simulink model "SPNCS_example_wx_timer"  (R2022b)
settings: Solver=VariableStepAuto  StartTime=0.0  StopTime=T  MaxStep=MaxStep  RelTol=RelTol
values from neighbouring files (symbols this model uses):
  epsilon = 0.0014    [initialization.m]
  J = 100000000    [initialization.m]
  rule = 2    [initialization.m]
  T = 20    [initialization.m]
  tau_mati = epsilon*T_star    (= 0.00123088)    [initialization.m]
  tau_miati = tau_mati    (= 0.00123088)    [initialization.m]
  tau_s_mati = 0.1072    [initialization.m]
  tau_s_miati = 0.0029    [initialization.m]
  x0 = [10;-2;5;0;0;0;0;0]    [initialization.m]
undefined symbols (not defined in the file or in its folder): tau_f_mati, tau_f_miati
libraries: simulink x6
settings Model: Creator=weixuanw  LastModifiedBy=weixuanw
settings ModelReferenceCC: EnableRefExpFcnMdlSchedulingChecks=on

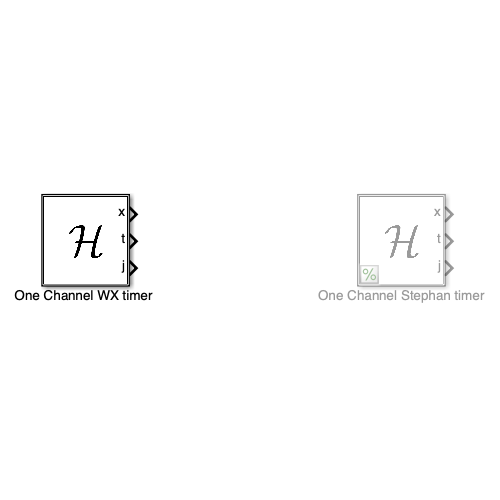
[thumbnail: Simulink's stored preview of the top-level diagram]
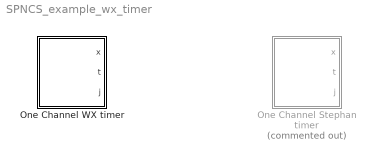
== system SPNCS_example_wx_timer ==
  One Channel Stephan timer : Subsystem  Commented=on  LoadFcn=set_param(gcb,'LinkStatus','none')
      settings: CopyFcn=|
      | set_param(gcb,'LinkStatus','none'),
      | set_param(gcs, 'MaxStep', 'MaxStep', 'RelTol', 'RelTol','Stop time', 'T')
      mask Display:
      | image(imread('Hcal.jpg'))
      | %plot([5 20 20 5 5],[5 5 20 20 5])
      | %text(8,13,'HyEq_mdl')
      | port_label('output', 1, 'x')
      | port_label('output', 2, 't')
      | port_label('output', 3, 'j')
  "One Channel WX timer " : Subsystem  LoadFcn=set_param(gcb,'LinkStatus','none')
      settings: CopyFcn=|
      | set_param(gcb,'LinkStatus','none'),
      | set_param(gcs, 'MaxStep', 'MaxStep', 'RelTol', 'RelTol','Stop time', 'T')
      mask Display:
      | image(imread('Hcal.jpg'))
      | %plot([5 20 20 5 5],[5 5 20 20 5])
      | %text(8,13,'HyEq_mdl')
      | port_label('output', 1, 'x')
      | port_label('output', 2, 't')
      | port_label('output', 3, 'j')

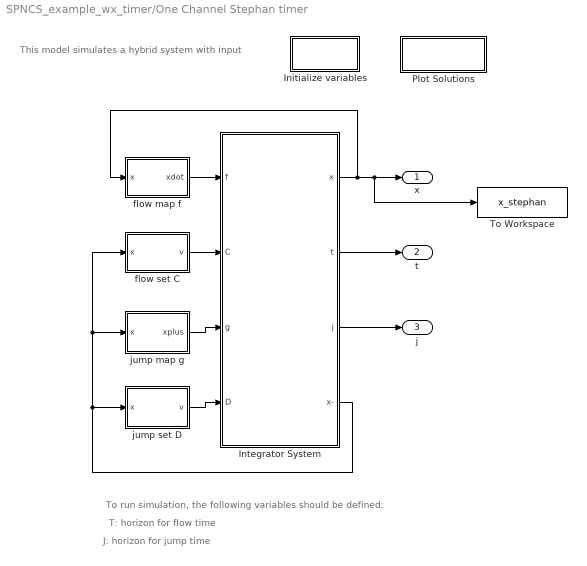
== system SPNCS_example_wx_timer/One Channel Stephan timer ==
  note: J: horizon for jump time
  note: T: horizon for flow time
  note: To run simulation, the following variables should be defined:
  note: This model simulates a hybrid system with input
  Initialize variables : Subsystem  Priority=-10
      settings: OpenFcn=|
      | try
      |      clearvars -except inifile pathfile_in pathfile_pos posfile
      |      cd(pathfile_in);
      |      eval(inifile);
      | catch
      |      [inifile,pathfile_in] = getInitializationfile;
      |      cd(pathfile_in);
      |      inifile = strrep(inifile,'.m','');
      |      eval(inifile);
      | end
      mask Display: disp('Double Click\n to Initialize')
  Integrator System : Subsystem  Priority=2  mask(Hybrid Integrator){T=T, J=J, x0=x0}
      mask prompts: T "Flow Horizon"; J "Jump Horizon"; x0 "Initial Condition"
      mask help:
      | This block integrates the state of the hybrid system defined by the flow map f (first input), the flow set C (second input), the jump map g (third input) and the jump set D (fourth input).
      | Starting from the initial condition x0 (last mask parameter), the system's state x evolves continuously within the set C, according to f(x,u), but is also subject to jumps within D, according to g(x,u).
      | The block also stops the simulation when the time t is greater than the flow horizon T (first mask parameter), or when the number of jumps j is greater than the jump horizon J (second mask parameter).
      | The outputs of the blocks are respectively x(t), t, j, x(t-).
      mask Help:
      | This block integrates the state of the hybrid system defined by the flow map f (first input), the flow set C (second input), the jump map g (third input) and the jump set D (fourth input).
      | <br>
      | Starting from the initial condition x0 (last mask parameter), the system's state x evolves continuously within the set C, according to f(x,u), but is also subject to jumps within D, according to g(x,u).
      | <br>
      | The block also stops the simulation when the time t is greater than the flow horizon T (first mask parameter), or when the number of jumps j is greater than the jump horizon J (second mask parameter).
      | <br>
      | The outputs of the blocks are respectively x(t), t, j, x(t-).
      | <br>
      | You can right click on the block and "Look under mask" to see what's inside the block.
      | Finally, refer to the manual (HybridSimulator_vXX.pdf) for more detailed information on how this hybrid simulator works.
  Plot Solutions : Subsystem
      settings: OpenFcn=|
      | try
      |      cd(pathfile_pos);
      |      eval(posfile);
      | catch
      |      [posfile,pathfile_pos] = getInitializationfile;
      |      cd(pathfile_pos);
      |      posfile = strrep(posfile,'.m','');
      |      eval(posfile);
      | end
      mask Display: disp('Double Click to\n Plot Solutions')
  To Workspace : ToWorkspace  VariableName=x_stephan  SampleTime=-1
  flow map f : MATLAB Function  TreatAsAtomicUnit=on
  flow set C : MATLAB Function  TreatAsAtomicUnit=on
  jump map g : MATLAB Function  Priority=2  TreatAsAtomicUnit=on
  jump set D : MATLAB Function  TreatAsAtomicUnit=on
  x : Outport
  t : Outport  Port=2
  j : Outport  Port=3
  wires:
  jump map g/1(xplus) -> Integrator System/3(g)
  jump set D/1(v) -> Integrator System/4(D)
  Integrator System/3(j) -> j/1
  Integrator System/2(t) -> t/1
  flow set C/1(v) -> Integrator System/2(C)
  Integrator System/1(x) -> To Workspace/1, x/1, flow map f/1(x)
  Integrator System/4(x-) -> flow set C/1(x), jump map g/1(x), jump set D/1(x)
  flow map f/1(xdot) -> Integrator System/1(f)

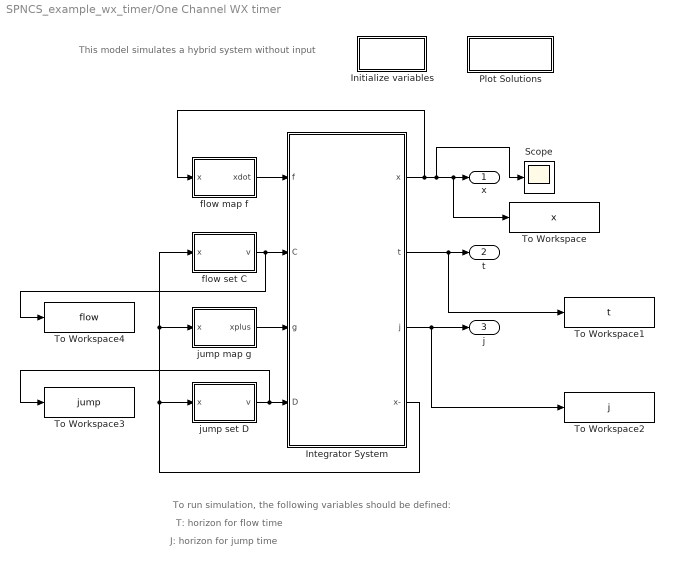
== system SPNCS_example_wx_timer/One Channel WX timer  ==
  note: J: horizon for jump time
  note: T: horizon for flow time
  note: To run simulation, the following variables should be defined:
  note: This model simulates a hybrid system without input
  Initialize variables : Subsystem  Priority=-10
      settings: OpenFcn=|
      | try
      |      clearvars -except inifile pathfile_in pathfile_pos posfile
      |      cd(pathfile_in);
      |      eval(inifile);
      | catch
      |      [inifile,pathfile_in] = getInitializationfile;
      |      cd(pathfile_in);
      |      inifile = strrep(inifile,'.m','');
      |      eval(inifile);
      | end
      mask Display: disp('Double Click\n to Initialize')
  Integrator System : Subsystem  Priority=2  mask(Hybrid Integrator){T=T, J=J, x0=x0}
      mask prompts: T "Flow Horizon"; J "Jump Horizon"; x0 "Initial Condition"
      mask help:
      | This block integrates the state of the hybrid system defined by the flow map f (first input), the flow set C (second input), the jump map g (third input) and the jump set D (fourth input).
      | Starting from the initial condition x0 (last mask parameter), the system's state x evolves continuously within the set C, according to f(x,u), but is also subject to jumps within D, according to g(x,u).
      | The block also stops the simulation when the time t is greater than the flow horizon T (first mask parameter), or when the number of jumps j is greater than the jump horizon J (second mask parameter).
      | The outputs of the blocks are respectively x(t), t, j, x(t-).
      mask Help:
      | This block integrates the state of the hybrid system defined by the flow map f (first input), the flow set C (second input), the jump map g (third input) and the jump set D (fourth input).
      | <br>
      | Starting from the initial condition x0 (last mask parameter), the system's state x evolves continuously within the set C, according to f(x,u), but is also subject to jumps within D, according to g(x,u).
      | <br>
      | The block also stops the simulation when the time t is greater than the flow horizon T (first mask parameter), or when the number of jumps j is greater than the jump horizon J (second mask parameter).
      | <br>
      | The outputs of the blocks are respectively x(t), t, j, x(t-).
      | <br>
      | You can right click on the block and "Look under mask" to see what's inside the block.
      | Finally, refer to the manual (HybridSimulator_vXX.pdf) for more detailed information on how this hybrid simulator works.
  Plot Solutions : Subsystem
      settings: OpenFcn=|
      | try
      |      cd(pathfile_pos);
      |      eval(posfile);
      | catch
      |      [posfile,pathfile_pos] = getInitializationfile;
      |      cd(pathfile_pos);
      |      posfile = strrep(posfile,'.m','');
      |      eval(posfile);
      | end
      mask Display: disp('Double Click to\n Plot Solutions')
  Scope : Scope
  To Workspace : ToWorkspace  VariableName=x  SampleTime=-1
  To Workspace1 : ToWorkspace  VariableName=t  SampleTime=-1
  To Workspace2 : ToWorkspace  VariableName=j  SampleTime=-1
  To Workspace3 : ToWorkspace  VariableName=jump  SampleTime=-1
  To Workspace4 : ToWorkspace  VariableName=flow  SampleTime=-1
  flow map f : MATLAB Function  TreatAsAtomicUnit=on
  flow set C : MATLAB Function  TreatAsAtomicUnit=on
  jump map g : MATLAB Function  Priority=2  TreatAsAtomicUnit=on
  jump set D : MATLAB Function  TreatAsAtomicUnit=on
  x : Outport
  t : Outport  Port=2
  j : Outport  Port=3
  wires:
  jump map g/1(xplus) -> Integrator System/3(g)
  jump set D/1(v) -> To Workspace3/1, Integrator System/4(D)
  Integrator System/3(j) -> To Workspace2/1, j/1
  Integrator System/2(t) -> To Workspace1/1, t/1
  flow set C/1(v) -> To Workspace4/1, Integrator System/2(C)
  Integrator System/1(x) -> Scope/1, To Workspace/1, x/1, flow map f/1(x)
  Integrator System/4(x-) -> flow set C/1(x), jump map g/1(x), jump set D/1(x)
  flow map f/1(xdot) -> Integrator System/1(f)

== system SPNCS_example_wx_timer/One Channel Stephan timer/Initialize variables ==

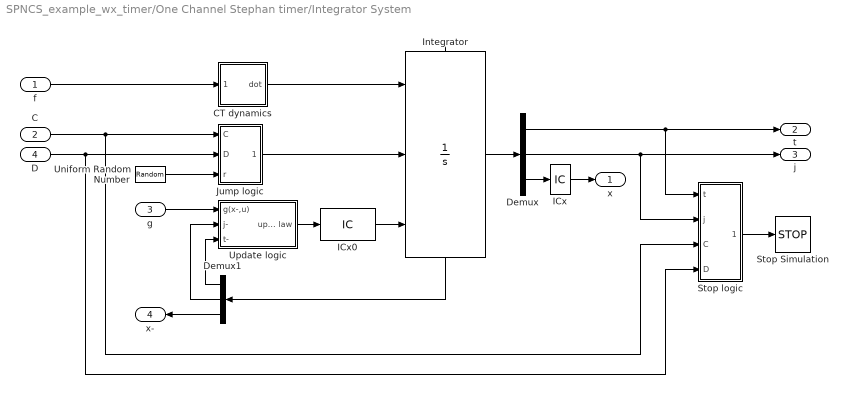
== system SPNCS_example_wx_timer/One Channel Stephan timer/Integrator System ==
  f : Inport
  C : Inport  Port=2
  g : Inport  Port=3
  D : Inport  Port=4
  CT dynamics : Subsystem
  Demux : Demux  Outputs=[1 1 -1]
  Demux1 : Demux  Outputs=[1 1 -1]
  ICx : InitialCondition  Value=x0
  ICx0 : InitialCondition  Value=[0; 0; x0(:)]
  Integrator : Integrator  ExternalReset=level hold  InitialConditionSource=external  ShowStatePort=on  ZeroCross=off
  Jump logic : Subsystem
  Stop Simulation : Stop
  Stop logic : Subsystem
  Uniform Random Number : UniformRandomNumber  Minimum=0  Seed=abs(floor(100*rand))  SampleTime=0
  Update logic : Subsystem
  x : Outport
  t : Outport  Port=2
  j : Outport  Port=3
  x- : Outport  Port=4
  wires:
  ICx0/1 -> Integrator/3
  ICx/1 -> x/1
  Demux/3 -> ICx/1
  Integrator/State -> Demux1/1
  Demux/2 -> j/1, Stop logic/2(j)
  Demux/1 -> t/1, Stop logic/1(t)
  Update logic/1(update law) -> ICx0/1
  CT dynamics/1(dot) -> Integrator/1
  Stop logic/1(stop) -> Stop Simulation/1
  Integrator/1 -> Demux/1
  C/1 -> Stop logic/3(C), Jump logic/1(C)
  D/1 -> Stop logic/4(D), Jump logic/2(D)
  f/1 -> CT dynamics/1(f(x,u))
  Demux1/3 -> x-/1
  Jump logic/1(jump) -> Integrator/2
  Uniform Random Number/1 -> Jump logic/3(r)
  g/1 -> Update logic/1(g(x-,u))
  Demux1/1 -> Update logic/3(t-)
  Demux1/2 -> Update logic/2(j-)

== system SPNCS_example_wx_timer/One Channel Stephan timer/Plot Solutions ==

== system SPNCS_example_wx_timer/One Channel WX timer /Initialize variables ==

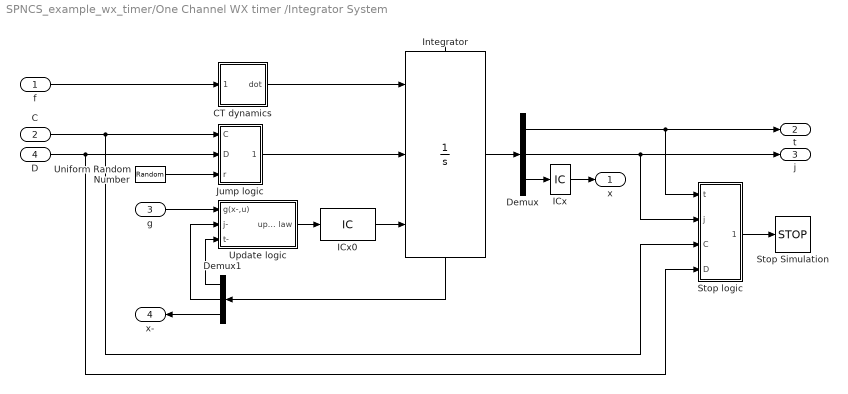
== system SPNCS_example_wx_timer/One Channel WX timer /Integrator System ==
  f : Inport
  C : Inport  Port=2
  g : Inport  Port=3
  D : Inport  Port=4
  CT dynamics : Subsystem
  Demux : Demux  Outputs=[1 1 -1]
  Demux1 : Demux  Outputs=[1 1 -1]
  ICx : InitialCondition  Value=x0
  ICx0 : InitialCondition  Value=[0; 0; x0(:)]
  Integrator : Integrator  ExternalReset=level hold  InitialConditionSource=external  ShowStatePort=on  ZeroCross=off
  Jump logic : Subsystem
  Stop Simulation : Stop
  Stop logic : Subsystem
  Uniform Random Number : UniformRandomNumber  Minimum=0  Seed=abs(floor(100*rand))  SampleTime=0
  Update logic : Subsystem
  x : Outport
  t : Outport  Port=2
  j : Outport  Port=3
  x- : Outport  Port=4
  wires:
  ICx0/1 -> Integrator/3
  ICx/1 -> x/1
  Demux/3 -> ICx/1
  Integrator/State -> Demux1/1
  Demux/2 -> j/1, Stop logic/2(j)
  Demux/1 -> t/1, Stop logic/1(t)
  Update logic/1(update law) -> ICx0/1
  CT dynamics/1(dot) -> Integrator/1
  Stop logic/1(stop) -> Stop Simulation/1
  Integrator/1 -> Demux/1
  C/1 -> Stop logic/3(C), Jump logic/1(C)
  D/1 -> Stop logic/4(D), Jump logic/2(D)
  f/1 -> CT dynamics/1(f(x,u))
  Demux1/3 -> x-/1
  Jump logic/1(jump) -> Integrator/2
  Uniform Random Number/1 -> Jump logic/3(r)
  g/1 -> Update logic/1(g(x-,u))
  Demux1/1 -> Update logic/3(t-)
  Demux1/2 -> Update logic/2(j-)

== system SPNCS_example_wx_timer/One Channel WX timer /Plot Solutions ==

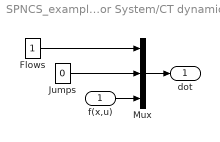
== system SPNCS_example_wx_timer/One Channel Stephan timer/Integrator System/CT dynamics ==
  f(x,u) : Inport
  Flows : Constant
  Jumps : Constant  Value=0
  Mux : Mux  Inputs=[1 1 -1]
  dot : Outport
  wires:
  Jumps/1 -> Mux/2
  Flows/1 -> Mux/1
  Mux/1 -> dot/1
  f(x,u)/1 -> Mux/3

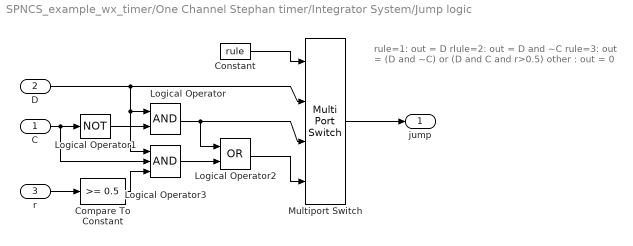
== system SPNCS_example_wx_timer/One Channel Stephan timer/Integrator System/Jump logic ==
  note: rule=1:  out = D
      | rlule=2: out = D and ~C
      | rule=3:  out = (D and ~C)  or (D and C and r>0.5)
      | other :  out = 0
  C : Inport
  D : Inport  Port=2
  r : Inport  Port=3
  Compare To Constant : simulink/Logic and Bit Operations/Compare To Constant  relop=>=  const=0.5  OutDataTypeStr=uint8
  Constant : Constant  Value=rule
  Logical Operator : Logic  AllPortsSameDT=off  OutDataTypeStr=boolean
  Logical Operator1 : Logic  Operator=NOT  Inputs=1  AllPortsSameDT=off  OutDataTypeStr=boolean
  Logical Operator2 : Logic  Operator=OR  AllPortsSameDT=off  OutDataTypeStr=boolean
  Logical Operator3 : Logic  Inputs=3  AllPortsSameDT=off  OutDataTypeStr=boolean
  Multiport Switch : MultiPortSwitch  SaturateOnIntegerOverflow=off  InputSameDT=off
  jump : Outport
  wires:
  Constant/1 -> Multiport Switch/1
  D/1 -> Logical Operator3/1, Logical Operator/1, Multiport Switch/2
  r/1 -> Compare To Constant/1
  C/1 -> Logical Operator3/2, Logical Operator1/1
  Logical Operator1/1 -> Logical Operator/2
  Logical Operator/1 -> Multiport Switch/3, Logical Operator2/1
  Logical Operator2/1 -> Multiport Switch/4
  Multiport Switch/1 -> jump/1
  Compare To Constant/1 -> Logical Operator3/3
  Logical Operator3/1 -> Logical Operator2/2

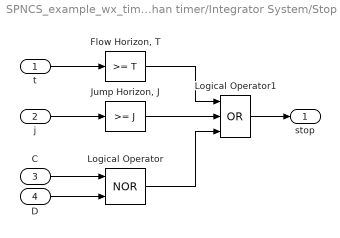
== system SPNCS_example_wx_timer/One Channel Stephan timer/Integrator System/Stop logic ==
  t : Inport
  j : Inport  Port=2
  C : Inport  Port=3
  D : Inport  Port=4
  "Flow Horizon, T" : simulink/Logic and Bit Operations/Compare To Constant  relop=>=  const=T  OutDataTypeStr=uint8  ZeroCross=off
  "Jump Horizon, J" : simulink/Logic and Bit Operations/Compare To Constant  relop=>=  const=J  OutDataTypeStr=uint8  ZeroCross=off
  Logical Operator : Logic  Operator=NOR  AllPortsSameDT=off  OutDataTypeStr=boolean
  Logical Operator1 : Logic  Operator=OR  Inputs=3  AllPortsSameDT=off  OutDataTypeStr=boolean
  stop : Outport
  wires:
  "Flow Horizon, T"/1 -> Logical Operator1/1
  "Jump Horizon, J"/1 -> Logical Operator1/2
  Logical Operator/1 -> Logical Operator1/3
  D/1 -> Logical Operator/2
  t/1 -> "Flow Horizon, T"/1
  j/1 -> "Jump Horizon, J"/1
  C/1 -> Logical Operator/1
  Logical Operator1/1 -> stop/1

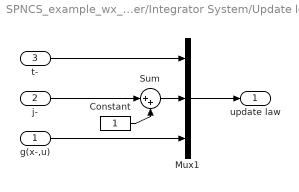
== system SPNCS_example_wx_timer/One Channel Stephan timer/Integrator System/Update logic ==
  g(x-,u) : Inport
  j- : Inport  Port=2
  t- : Inport  Port=3
  Constant : Constant
  Mux1 : Mux  Inputs=[1 1 -1]
  Sum : Sum  Inputs=|++
  update law : Outport
  wires:
  Sum/1 -> Mux1/2
  Mux1/1 -> update law/1
  j-/1 -> Sum/1
  g(x-,u)/1 -> Mux1/3
  t-/1 -> Mux1/1
  Constant/1 -> Sum/2

== system SPNCS_example_wx_timer/One Channel WX timer /Integrator System/CT dynamics ==
  f(x,u) : Inport
  Flows : Constant
  Jumps : Constant  Value=0
  Mux : Mux  Inputs=[1 1 -1]
  dot : Outport
  wires:
  Jumps/1 -> Mux/2
  Flows/1 -> Mux/1
  Mux/1 -> dot/1
  f(x,u)/1 -> Mux/3

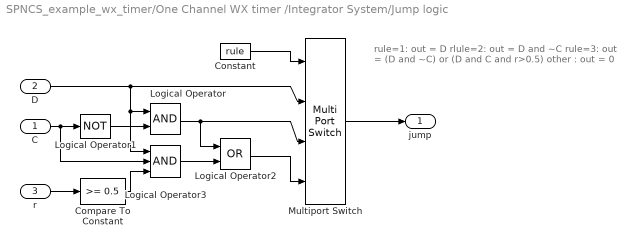
== system SPNCS_example_wx_timer/One Channel WX timer /Integrator System/Jump logic ==
  note: rule=1:  out = D
      | rlule=2: out = D and ~C
      | rule=3:  out = (D and ~C)  or (D and C and r>0.5)
      | other :  out = 0
  C : Inport
  D : Inport  Port=2
  r : Inport  Port=3
  Compare To Constant : simulink/Logic and Bit Operations/Compare To Constant  relop=>=  const=0.5  OutDataTypeStr=uint8
  Constant : Constant  Value=rule
  Logical Operator : Logic  AllPortsSameDT=off  OutDataTypeStr=boolean
  Logical Operator1 : Logic  Operator=NOT  Inputs=1  AllPortsSameDT=off  OutDataTypeStr=boolean
  Logical Operator2 : Logic  Operator=OR  AllPortsSameDT=off  OutDataTypeStr=boolean
  Logical Operator3 : Logic  Inputs=3  AllPortsSameDT=off  OutDataTypeStr=boolean
  Multiport Switch : MultiPortSwitch  SaturateOnIntegerOverflow=off  InputSameDT=off
  jump : Outport
  wires:
  Constant/1 -> Multiport Switch/1
  D/1 -> Logical Operator3/1, Logical Operator/1, Multiport Switch/2
  r/1 -> Compare To Constant/1
  C/1 -> Logical Operator3/2, Logical Operator1/1
  Logical Operator1/1 -> Logical Operator/2
  Logical Operator/1 -> Multiport Switch/3, Logical Operator2/1
  Logical Operator2/1 -> Multiport Switch/4
  Multiport Switch/1 -> jump/1
  Compare To Constant/1 -> Logical Operator3/3
  Logical Operator3/1 -> Logical Operator2/2

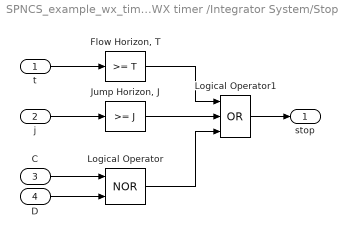
== system SPNCS_example_wx_timer/One Channel WX timer /Integrator System/Stop logic ==
  t : Inport
  j : Inport  Port=2
  C : Inport  Port=3
  D : Inport  Port=4
  "Flow Horizon, T" : simulink/Logic and Bit Operations/Compare To Constant  relop=>=  const=T  OutDataTypeStr=uint8  ZeroCross=off
  "Jump Horizon, J" : simulink/Logic and Bit Operations/Compare To Constant  relop=>=  const=J  OutDataTypeStr=uint8  ZeroCross=off
  Logical Operator : Logic  Operator=NOR  AllPortsSameDT=off  OutDataTypeStr=boolean
  Logical Operator1 : Logic  Operator=OR  Inputs=3  AllPortsSameDT=off  OutDataTypeStr=boolean
  stop : Outport
  wires:
  "Flow Horizon, T"/1 -> Logical Operator1/1
  "Jump Horizon, J"/1 -> Logical Operator1/2
  Logical Operator/1 -> Logical Operator1/3
  D/1 -> Logical Operator/2
  t/1 -> "Flow Horizon, T"/1
  j/1 -> "Jump Horizon, J"/1
  C/1 -> Logical Operator/1
  Logical Operator1/1 -> stop/1

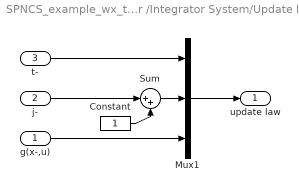
== system SPNCS_example_wx_timer/One Channel WX timer /Integrator System/Update logic ==
  g(x-,u) : Inport
  j- : Inport  Port=2
  t- : Inport  Port=3
  Constant : Constant
  Mux1 : Mux  Inputs=[1 1 -1]
  Sum : Sum  Inputs=|++
  update law : Outport
  wires:
  Sum/1 -> Mux1/2
  Mux1/1 -> update law/1
  j-/1 -> Sum/1
  g(x-,u)/1 -> Mux1/3
  t-/1 -> Mux1/1
  Constant/1 -> Sum/2

== matlab function SPNCS_example_wx_timer/One Channel Stephan timer/flow map f ==
  data: x input; xdot output; epsilon parameter
function xdot = f(x, epsilon)
% x = [x1; x2; z; e_x; e_z; tau_s; tau_f]
xtemp = x;

x1 = xtemp(1);
x2 = xtemp(2);
z  = xtemp(3);
e_x = xtemp(4);
e_z = xtemp(5);
tau_s = xtemp(6);
tau_f = xtemp(7);

x1_dot = x2;
x2_dot = z;
z_dot  = (1/epsilon)*(- x1 - x2 - z - e_x - e_z);

e_x_dot = -z;
e_z_dot = (1/epsilon)*(x1 + x2 + z + e_x + e_z);
tau_s_dot = 1;
tau_f_dot = 1/epsilon;

xdot = [x1_dot; x2_dot; z_dot; e_x_dot; e_z_dot; tau_s_dot; tau_f_dot];

== matlab function SPNCS_example_wx_timer/One Channel Stephan timer/flow set C ==
  data: x input; v output; tau_s_mati parameter; tau_f_mati parameter; epsilon parameter; tau_s_miati parameter; tau_f_miati parameter
function v  = C(x, tau_s_mati, tau_f_mati, epsilon, tau_s_miati, tau_f_miati) 

% Check on flow conditions
% E.g.,
% if (x(1) >= u(1))  % flow condition
%     v = 1;  % report flow
% else
%     v = 0;   % do not report flow
% end

% x = [x1; x2; z; e_x; e_z; tau_s; tau_f]
xtemp = x;

x1 = xtemp(1);
x2 = xtemp(2);
z  = xtemp(3);
e_x = xtemp(4);
e_z = xtemp(5);
tau_s = xtemp(6);
tau_f = xtemp(7);


Ds_st = (tau_s_miati <= tau_s) && ...
        (tau_f_miati <= epsilon*tau_f) && (epsilon*tau_f <= tau_f_mati-tau_f_miati);

Df_st = (tau_f_miati <= epsilon*tau_f) && ...
        (tau_f_miati <= tau_s) && (tau_s <= tau_s_mati-tau_f_miati);

squre = (tau_s_mati-tau_f_miati <= tau_s) && (tau_s <= tau_s_mati) && ...
        (tau_f_mati-tau_f_miati <= epsilon*tau_f) && (epsilon*tau_f <= tau_f_mati);

C_st = (0 <= epsilon*tau_f) && (epsilon*tau_f <= tau_f_mati) && ...
       (0 <= tau_s) && (tau_s <= tau_s_mati) && ...
       (~squre);

%%%%%%%%%%%%%%%%%%%%%%%%%%%%%%%%%%%
if C_st
    v = 1;
else
    v = 0;
end

== matlab function SPNCS_example_wx_timer/One Channel Stephan timer/jump map g ==
  data: x input; xplus output; tau_s_miati parameter; tau_s_mati parameter; tau_f_miati parameter; tau_f_mati parameter; epsilon parameter
function xplus = g(x, tau_s_miati, tau_s_mati, tau_f_miati, tau_f_mati, epsilon)

xtemp = x;

x1 = xtemp(1);
x2 = xtemp(2);
z  = xtemp(3);
e_x = xtemp(4);
e_z = xtemp(5);
tau_s = xtemp(6);
tau_f = xtemp(7);

x1_plus = x1;
x2_plus = x2;
z_plus = z;
e_x_plus = e_x;
e_z_plus = e_z;
tau_s_plus = tau_s;
tau_f_plus = tau_f;

% Since we want to reduce the total number of jumps, we give fast update a 
% higher priority. So we first check if we are in Df, if yes, we do fast
% jump.
Ds_st = (tau_s_miati <= tau_s) && ...
        (tau_f_miati <= epsilon*tau_f) && (epsilon*tau_f <= tau_f_mati-tau_f_miati);

Df_st = (tau_f_miati <= epsilon*tau_f) && ...
        (tau_f_miati <= tau_s) && (tau_s <= tau_s_mati-tau_f_miati);


if Df_st % If we are in Df, we do fast jump

    x1_plus = x1;
    x2_plus = x2;
    z_plus = z;
    e_x_plus = e_x;
    e_z_plus = 0;
    tau_s_plus = tau_s;
    tau_f_plus = 0;
    
else % If we are not in Df, we must in Ds, we do slow jump
    x1_plus = x1;
    x2_plus = x2;
    z_plus = z;
    e_x_plus = 0;
    e_z_plus = e_z;
    tau_s_plus = 0;
    tau_f_plus = tau_f; 
    
end

xplus = [x1_plus; x2_plus; z_plus; e_x_plus; e_z_plus; tau_s_plus; tau_f_plus];

== matlab function SPNCS_example_wx_timer/One Channel Stephan timer/jump set D ==
  data: x input; v output; tau_s_miati parameter; tau_s_mati parameter; tau_f_miati parameter; tau_f_mati parameter; epsilon parameter
function v  = D(x, tau_s_miati, tau_s_mati, tau_f_miati, tau_f_mati, epsilon) 


xtemp = x;

x1 = xtemp(1);
x2 = xtemp(2);
z  = xtemp(3);
e_x = xtemp(4);
e_z = xtemp(5);
tau_s = xtemp(6);
tau_f = xtemp(7);

% Ds_wx = (tau_s_miati <= tau_s) && (tau_f_miati <= epsilon*tau_f);
% Df_wx = (tau_f_miati <= tau_s) && (tau_s <= tau_s_mati-tau_f_miati) && (tau_f_miati <= epsilon*tau_f);

Ds_st = (tau_s_miati <= tau_s) && ...
        (tau_f_miati <= epsilon*tau_f) && (epsilon*tau_f <= tau_f_mati-tau_f_miati);

Df_st = (tau_f_miati <= epsilon*tau_f) && ...
        (tau_f_miati <= tau_s) && (tau_s <= tau_s_mati-tau_f_miati);



if Ds_st || Df_st
    v = 1; % report jump
else
    v = 0;
end

== matlab function SPNCS_example_wx_timer/One Channel WX timer /flow map f ==
  data: x input; xdot output; epsilon parameter
function xdot = f(x, epsilon)
% x = [x_p; x_c; z_1; z_2; e_s; e_f; tau_s; tau]
xtemp = x;

x_p = xtemp(1);
x_c = xtemp(2);
z_1 = xtemp(3);
z_2 = xtemp(4);
e_s = xtemp(5);
e_f = xtemp(6);
tau_s = xtemp(7);
tau = xtemp(8);

a = 2.36;
k = 0.75;

x_p_dot = x_p + z_1 + 2*(-k*x_c+e_s);
x_c_dot = -a*x_c + a*(x_p+z_2+e_f);
z_1_dot = (1/epsilon)*(-z_1 + k*x_c - e_s);
z_2_dot = (1/epsilon)*(x_p - z_1 - z_2 + k*x_c - e_s);

e_s_dot = -a*k*x_c + a*k*(x_p+z_2+e_f);
e_f_dot = -(1/epsilon)*(x_p + z_1 - 2*k*x_c + e_s) - (x_p - z_1 - z_2 + k*x_c - e_s);

tau_s_dot = 1;
tau_dot = 1/epsilon;

xdot = [x_p_dot; x_c_dot; z_1_dot; z_2_dot; e_s_dot; e_f_dot; tau_s_dot; tau_dot];

== matlab function SPNCS_example_wx_timer/One Channel WX timer /flow set C ==
  data: x input; v output; tau_s_mati parameter; tau_mati parameter; epsilon parameter
function v  = C(x, tau_s_mati, tau_mati, epsilon) 

% Check on flow conditions
% E.g.,
% if (x(1) >= u(1))  % flow condition
%     v = 1;  % report flow
% else
%     v = 0;   % do not report flow
% end

% x = [x_p; x_c; z_1; z_2; e_s; e_f; tau_s; tau]
xtemp = x;

x_p = xtemp(1);
x_c = xtemp(2);
z_1 = xtemp(3);
z_2 = xtemp(4);
e_s = xtemp(5);
e_f = xtemp(6);
tau_s = xtemp(7);
tau = xtemp(8);


%%%%%%%%%%%%%%%%%%%%%%%%%%%%%%%%%%%
if ((0 <= tau_s)&&(tau_s < tau_s_mati)&& ...
        (0 <= epsilon*tau)&&(epsilon*tau < tau_mati))
    v = 1;
else
    v = 0;
end

== matlab function SPNCS_example_wx_timer/One Channel WX timer /jump map g ==
  data: x input; xplus output; tau_s_miati parameter; tau_s_mati parameter; tau_miati parameter; tau_mati parameter; epsilon parameter
function xplus = g(x, tau_s_miati, tau_s_mati, tau_miati, tau_mati, epsilon)

% x = [x_p; x_c; z_1; z_2; e_s; e_f; tau_s; tau]
xtemp = x;

x_p = xtemp(1);
x_c = xtemp(2);
z_1 = xtemp(3);
z_2 = xtemp(4);
e_s = xtemp(5);
e_f = xtemp(6);
tau_s = xtemp(7);
tau = xtemp(8);


x_p_plus = x_p;
x_c_plus = x_c;
z_1_plus = z_1;
z_2_plus = z_2;
e_s_plus = e_s;
e_f_plus = e_f;
tau_s_plus = tau_s;
tau_plus = tau;

% Since we want to reduce the total number of jumps, we give fast update a 
% higher priority. So we first check if we are in Df, if yes, we do fast
% jump.
Df_wx = (tau_miati <= tau_s) && (tau_s <= tau_s_mati-tau_miati) && (tau_miati <= epsilon*tau);



if Df_wx % If we are in Df, we do fast jump

    x_p_plus = x_p;
    x_c_plus = x_c;
    z_1_plus = z_1;
    z_2_plus = z_2;
    e_s_plus = e_s;
    e_f_plus = 0;
    tau_s_plus = tau_s;
    tau_plus = 0;
else % If we are not in Df, we must in Ds, we do slow jump
    x_p_plus = x_p;
    x_c_plus = x_c;
    z_1_plus = z_1;
    z_2_plus = z_2;
    e_s_plus = 0;
    e_f_plus = e_f;
    tau_s_plus = 0;
    tau_plus = 0;
 % In slow update, both timers reset to zero.
    
end

xplus = [x_p_plus; x_c_plus; z_1_plus; z_2_plus; e_s_plus; e_f_plus; tau_s_plus;tau_plus];

== matlab function SPNCS_example_wx_timer/One Channel WX timer /jump set D ==
  data: x input; v output; tau_s_miati parameter; tau_s_mati parameter; tau_miati parameter; tau_mati parameter; epsilon parameter
function v  = D(x, tau_s_miati, tau_s_mati, tau_miati, tau_mati, epsilon) 

% x = [x_p; x_c; z_1; z_2; e_s; e_f; tau_s; tau]
xtemp = x;

x_p = xtemp(1);
x_c = xtemp(2);
z_1 = xtemp(3);
z_2 = xtemp(4);
e_s = xtemp(5);
e_f = xtemp(6);
tau_s = xtemp(7);
tau = xtemp(8);

% We do not write upperbound of jump set to avoid numerical error in
% MATLAB.
Ds_wx = (tau_s_miati <= tau_s) && (tau_miati <= epsilon*tau); 
Df_wx = (tau_miati <= tau_s) && (tau_s <= tau_s_mati-tau_miati) && (tau_miati <= epsilon*tau);



if Ds_wx || Df_wx
    v = 1; % report jump
else
    v = 0;
end
